simulink library "ilcPerfIndx_cl"  (R2018b)
settings: Solver=VariableStepAuto  StartTime=0.0  StopTime=10.0  RelTol=1e-3
libraries: stopwatch_ul x2, runningAvg_ul x1
settings Model: Creator=mcobb  LastModifiedBy=mcobb

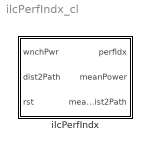
== system ilcPerfIndx_cl ==
  ilcPerfIndx : Subsystem  mask{w=0}
      mask prompts: w "Distance Penalty Weight"

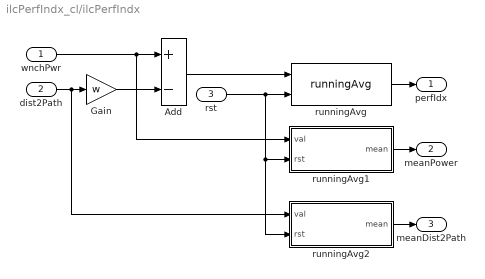
== system ilcPerfIndx_cl/ilcPerfIndx ==
  wnchPwr : Inport  PortDimensions=1
  dist2Path : Inport  Port=2  PortDimensions=1
  rst : Inport  Port=3  PortDimensions=1
  Add : Sum  Inputs=+-
  Gain : Gain  Gain=w
  runningAvg : runningAvg_ul/runningAvg  SystemSampleTime=-1
  runningAvg1 : Subsystem
  runningAvg2 : Subsystem
  perfIdx : Outport  PortDimensions=1
  meanPower : Outport  Port=2  PortDimensions=1
  meanDist2Path : Outport  Port=3  PortDimensions=1
  wires:
  Gain/1 -> Add/2
  wnchPwr/1 -> runningAvg1/1(val), Add/1
  dist2Path/1 -> runningAvg2/1(val), Gain/1
  rst/1 -> runningAvg2/2(rst), runningAvg1/2(rst), runningAvg/2
  Add/1 -> runningAvg/1
  runningAvg/1 -> perfIdx/1
  runningAvg1/1(mean) -> meanPower/1
  runningAvg2/1(mean) -> meanDist2Path/1

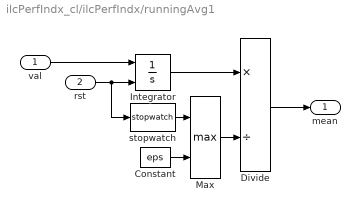
== system ilcPerfIndx_cl/ilcPerfIndx/runningAvg1 ==
  val : Inport
  rst : Inport  Port=2
  Constant : Constant  Value=eps
  Divide : Product  Inputs=*/
  Integrator : Integrator  ExternalReset=rising
  Max : MinMax  Function=max  Inputs=2
  stopwatch : stopwatch_ul/stopwatch  SystemSampleTime=-1
  mean : Outport
  wires:
  Integrator/1 -> Divide/1
  val/1 -> Integrator/1
  stopwatch/1 -> Max/1
  Divide/1 -> mean/1
  Constant/1 -> Max/2
  Max/1 -> Divide/2
  rst/1 -> stopwatch/1, Integrator/2

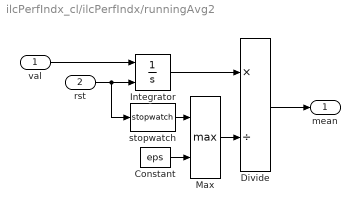
== system ilcPerfIndx_cl/ilcPerfIndx/runningAvg2 ==
  val : Inport
  rst : Inport  Port=2
  Constant : Constant  Value=eps
  Divide : Product  Inputs=*/
  Integrator : Integrator  ExternalReset=rising
  Max : MinMax  Function=max  Inputs=2
  stopwatch : stopwatch_ul/stopwatch  SystemSampleTime=-1
  mean : Outport
  wires:
  rst/1 -> Integrator/2, stopwatch/1
  Max/1 -> Divide/2
  Constant/1 -> Max/2
  Divide/1 -> mean/1
  stopwatch/1 -> Max/1
  val/1 -> Integrator/1
  Integrator/1 -> Divide/1
